simulink model "lqr"  (Simulink 7.4)
settings: Solver=FixedStepDiscrete  StartTime=0.0  StopTime=20  FixedStep=0.005  RelTol=1e-3
settings Model: Creator=NGUYEN VINH HAO  LastModifiedBy=Admin
settings OptimizationCC: OptimizeModelRefInitCode=on  LifeSpan=1
settings RTWCC: SystemTargetFile=ert.tlc  GenCodeOnly=on  GenerateMakefile=off  TemplateMakefile=ert_default_tmf  Description=Real-Time Workshop Embedded Coder  ProcessScript=ert_make_rtw_hook
settings CodeAppCC: IgnoreCustomStorageClasses=off
settings ERTTargetCC: MultiwordLength=2048  GenerateSampleERTMain=on  ERTCustomFileTemplate=example_file_process.tlc  ConvertIfToSwitch=off

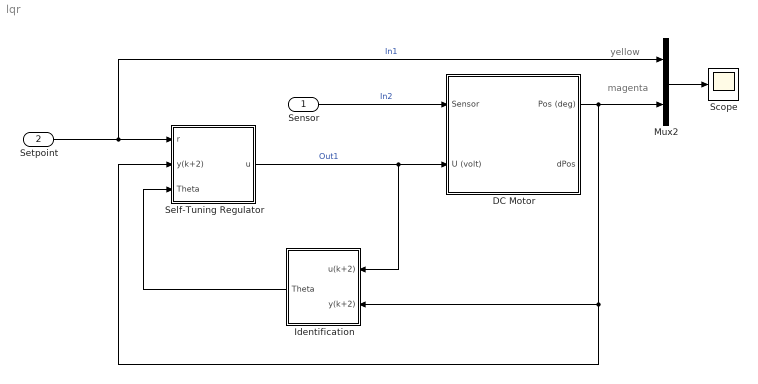
== system lqr ==
  note: yellow
  note: magenta
  Sensor : Inport  PortDimensions=1  OutDataType=sfix(16)  OutScaling=2^0
  Setpoint : Inport  Port=2  PortDimensions=1  OutDataType=sfix(16)  OutScaling=2^0
  DC Motor : Subsystem
  Identification : Subsystem
  Mux2 : Mux  Inputs=2
  Scope : Scope
      settings: YMin=1999.78  YMax=2000.03
  Self-Tuning Regulator : Subsystem
  wires:
  Sensor/1 -> DC Motor/1(Sensor)  "In2"
  Self-Tuning Regulator/1(u) -> DC Motor/2(U (volt)), Identification/1(u(k+2))  "Out1"
  Mux2/1 -> Scope/1
  Identification/1(Theta) -> Self-Tuning Regulator/3(Theta)
  Setpoint/1 -> Mux2/1, Self-Tuning Regulator/1(r)  "In1"
  DC Motor/1(Pos (deg)) -> Mux2/2, Identification/2(y(k+2)), Self-Tuning Regulator/2(y(k+2))

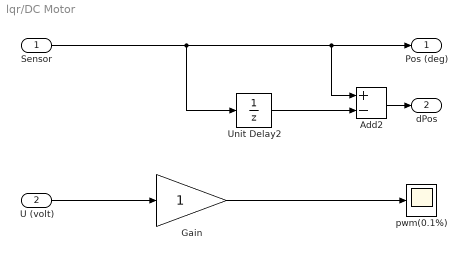
== system lqr/DC Motor ==
  Sensor : Inport  PortDimensions=1  OutDataType=sfix(16)  OutScaling=2^0
  U (volt) : Inport  Port=2  PortDimensions=1  OutDataType=sfix(16)  OutScaling=2^0
  Add2 : Sum  Inputs=+-  OutDataType=sfix(16)  OutScaling=2^-10
  Gain : Gain  ParameterDataType=sfix(16)  ParameterScaling=2^0  OutDataType=sfix(16)  OutScaling=2^0  ParamDataTypeStr=Inherit: Same as input
  Unit Delay2 : UnitDelay  SampleTime=-1
  pwm(0.1%) : Scope
      settings: YMin=-1100  YMax=1100  SaveName=ScopeData3  DataFormat=Array
  Pos (deg) : Outport  PortDimensions=1  OutDataType=sfix(16)  OutScaling=2^0
  dPos : Outport  Port=2  PortDimensions=1  OutDataType=sfix(16)  OutScaling=2^0
  wires:
  Unit Delay2/1 -> Add2/2
  Add2/1 -> dPos/1
  U (volt)/1 -> Gain/1
  Sensor/1 -> Add2/1, Pos (deg)/1, Unit Delay2/1
  Gain/1 -> pwm(0.1%)/1

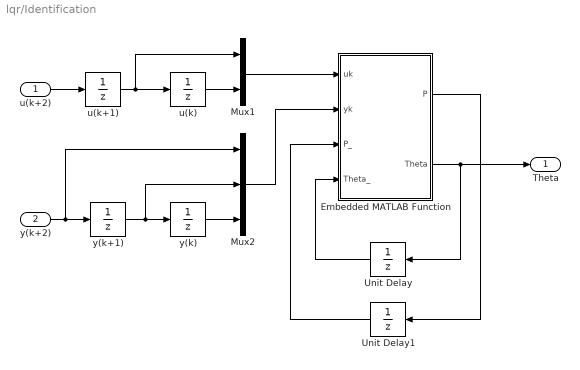
== system lqr/Identification ==
  u(k+2) : Inport  PortDimensions=1  OutDataType=fixdt(1, 16)  OutScaling=2^0
  y(k+2) : Inport  Port=2  PortDimensions=1  OutDataType=fixdt(1, 16)  OutScaling=2^0
  Embedded MATLAB Function : Stateflow chart
  Mux1 : Mux  Inputs=2
  Mux2 : Mux  Inputs=3
  Unit Delay : UnitDelay  X0=[-1; 0.1; 0.1; 1]  SampleTime=-1
  Unit Delay1 : UnitDelay  X0=1e5*eye(4)  SampleTime=-1
  u(k) : UnitDelay  SampleTime=-1
  u(k+1) : UnitDelay  SampleTime=-1
  y(k) : UnitDelay  SampleTime=-1
  y(k+1) : UnitDelay  SampleTime=-1
  Theta : Outport  PortDimensions=4  OutDataType=fixdt(1, 16)  OutScaling=2^0
  wires:
  Unit Delay/1 -> Embedded MATLAB Function/4(Theta_)
  Embedded MATLAB Function/2(Theta) -> Unit Delay/1, Theta/1
  Unit Delay1/1 -> Embedded MATLAB Function/3(P_)
  Embedded MATLAB Function/1(P) -> Unit Delay1/1
  Mux1/1 -> Embedded MATLAB Function/1(uk)
  y(k+1)/1 -> Mux2/2, y(k)/1
  y(k)/1 -> Mux2/3
  Mux2/1 -> Embedded MATLAB Function/2(yk)
  u(k)/1 -> Mux1/2
  u(k+1)/1 -> u(k)/1, Mux1/1
  u(k+2)/1 -> u(k+1)/1
  y(k+2)/1 -> y(k+1)/1, Mux2/1

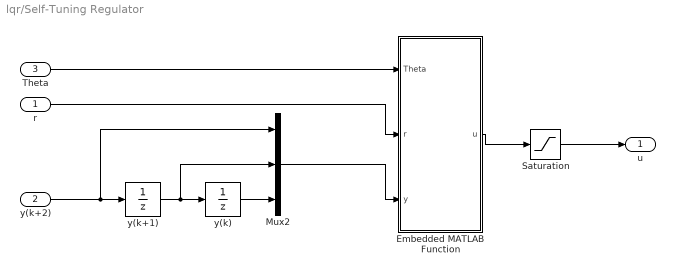
== system lqr/Self-Tuning Regulator ==
  r : Inport  PortDimensions=1  OutDataType=fixdt(1, 16)  OutScaling=2^0
  y(k+2) : Inport  Port=2  PortDimensions=1  OutDataType=fixdt(1, 16)  OutScaling=2^0
  Theta : Inport  Port=3  PortDimensions=4  OutDataType=sfix(16)  OutScaling=2^0
  Embedded MATLAB Function : Stateflow chart
  Mux2 : Mux  Inputs=3
  Saturation : Saturate  UpperLimit=12  LowerLimit=-12  OutDataType=fixdt(1, 16)  OutScaling=2^0
  y(k) : UnitDelay  SampleTime=-1
  y(k+1) : UnitDelay  SampleTime=-1
  u : Outport  PortDimensions=1  OutDataType=fixdt(1, 16)  OutScaling=2^0
  wires:
  r/1 -> Embedded MATLAB Function/2(r)
  Mux2/1 -> Embedded MATLAB Function/3(y)
  Theta/1 -> Embedded MATLAB Function/1(Theta)
  y(k+2)/1 -> Mux2/1, y(k+1)/1
  y(k)/1 -> Mux2/3
  y(k+1)/1 -> y(k)/1, Mux2/2
  Saturation/1 -> u/1
  Embedded MATLAB Function/1(u) -> Saturation/1

== matlab function Identification/Embedded MATLAB Function ==
  settings: fimath=|
      | fimath(...
      | 'RoundMode', 'floor',...
      | 'OverflowMode', 'wrap',...
      | 'ProductMode', 'KeepLSB', 'ProductWordLength', 32,...
      | 'SumMode', 'KeepLSB', 'SumWordLength', 32,...
      | 'CastBeforeSum', false)
  data: P output double; uk input double; yk input double; P_ input double; Theta_ input double; Theta output double
function [P,Theta] = Uocluong(uk,yk,P_,Theta_)

lamda = 0.95;
PHI = [-yk(2); -yk(3); uk(1); uk(2)];
e = yk(1) - PHI'*Theta_;
L = P_*PHI/(lamda+PHI'*P_*PHI);
P = 1/lamda*(P_-(P_*PHI)*(PHI'*P_)/(lamda+PHI'*P_*PHI));
Theta = Theta_ + L*e;

== matlab function Self-Tuning Regulator/Embedded MATLAB Function ==
  settings: fimath=|
      | fimath(...
      | 'RoundMode', 'floor',...
      | 'OverflowMode', 'wrap',...
      | 'ProductMode', 'KeepLSB', 'ProductWordLength', 32,...
      | 'SumMode', 'KeepLSB', 'SumWordLength', 32,...
      | 'CastBeforeSum', false)
  data: Theta input double; r input double; y input double; u output double
function u = LQR_pp1(Theta,r,y)
% Gan lai cho de su dung
a1 = Theta(1);
a2 = Theta(2);
b1 = Theta(3);
b2 = Theta(4);
% PT sai phan:
%     a0.z^2+a1.y.z+a2.y = b1.u.z + b2.u
% <=> y(k+2) + a1.y(k+1) + a2.y(k) = b1.u(k+1) + b2.u(k)
% PT Trang thai mo ta he thong tinh tu PT sai phan
% x(k+1) = Ad.x(k) + Bd.u(k)
% y(k) = Cd.x(k)
% Refer to Chuong 7 CSTD
beta1 = b1;
beta2 = (b2-a1*beta1);
Ad = [0 1; -a2 -a1];
Bd = [beta1; beta2];
Cd = [1 0];
x = [y(3); (y(2)-beta1*r)];
% LQR:
Q = [2 0;0 1];
R = 1;
I = eye(size(Ad));
P = eye(size(Ad));
E = Bd*R^-1*Bd';
while(1)
    P_ins = P ;
    P =  Ad'*P*((I+E*P)^-1)*Ad+Q;
    K = P-P_ins;
    if((abs(K(1)) < 10^-3) && (abs(K(2)) < 10^-3) && (abs(K(3)) < 10^-3) && (abs(K(4)) < 10^-3))
        break;
    end
end
L = (R^-1)*Bd'*(Ad^-1)'*(P-Q);
% Luat dieu khien
u = -L*x;
